simulink model "MySusp_StabiSystem_RTW"  (Simulink 10.3)
settings: Solver=ode1  StartTime=0.0  StopTime=inf  FixedStep=0.001  RelTol=1e-3
PreLoadFcn:
  | vehicle = 'Car'; if ~length(which('cmself')), cmenv; end
  | MySusp_StabiSystem_RTW_bus
  | MySusp_StabiSystem_RTW_params
InitFcn:
  | vehicle = 'Car'; if ~length(which('cmself')), cmenv; end
  | MySusp_StabiSystem_RTW_bus
undefined symbols (not defined in the file): Stiffness_F, Stiffness_R
Description:
  | CarMaker Plug-in Model Target
settings Model: Creator=ml  ModifiedByFormat=IPG  LastModifiedBy=IPG  MultithreadedSim=on
settings DataIOCC: SaveFormat=Dataset  SignalLoggingSaveFormat=Dataset  ReturnWorkspaceOutputs=on
settings OptimizationCC: ExpressionDepthLimit=128  LifeSpan=auto
settings DebuggingCC: UnderspecifiedInitializationDetection=Simplified  MergeDetectMultiDrivingBlocksExec=error  FcnCallInpInsideContextMsg=error  StateNameClashWarn=none  SFUnexpectedBacktrackingDiag=error  SFNoUnconditionalDefaultTransitionDiag=error  SFExecutionAtInitializationDiag=warning  SFMachineParentedDataDiag=error  ArithmeticOperatorsInVariantConditions=error
settings HardwareCC: ProdBitPerPointer=64  ProdBitPerSizeT=64  ProdBitPerPtrDiffT=64  ProdLargestAtomicFloat=Float  ProdIntDivRoundTo=Zero  ProdEndianess=LittleEndian  ProdWordSize=64  ProdHWDeviceType=Intel->x86-64 (Windows64)
settings ModelReferenceCC: PropagateSignalLabelsOutOfModel=on
settings SFSimCC: SimUseLocalCustomCode=on  CustomCodeUndefinedFunction=FilterOut
settings RTWCC: Description=CarMaker Plug-in Model Target  SystemTargetFile=CarMaker.tlc  TemplateMakefile=CarMaker_unix-win64.tmf  RTWUseLocalCustomCode=on
settings CodeAppCC: MaxIdLength=127  StateflowObjectComments=off
settings STFCustomTargetCC: TargetLangStandard=C99 (ISO)  CombineOutputUpdateFcns=on  MatFileLogging=on  CodeInterfacePackaging=Reusable function  GRTInterface=off  GenerateAllocFcn=on  SystemTargetFile=CarMaker.tlc
settings GRTTargetCC: TargetLangStandard=C99 (ISO)  ParMdlRefBuildCompliant=off  CompOptLevelCompliant=off  ConcurrentExecutionCompliant=off  CombineOutputUpdateFcns=on  CodeInterfacePackaging=Reusable function  CPPClassGenCompliant=off  GRTInterface=off  GenerateAllocFcn=on  UseToolchainInfoCompliant=off
settings CustomProperty: DataType=string
settings EnumStrPairs: String=Car
settings ConfigComp: CovMetricSettings=dwe  CovSaveCumulativeToWorkspaceVar=off  CovSaveSingleToWorkspaceVar=off  CovExternalEMLEnable=on

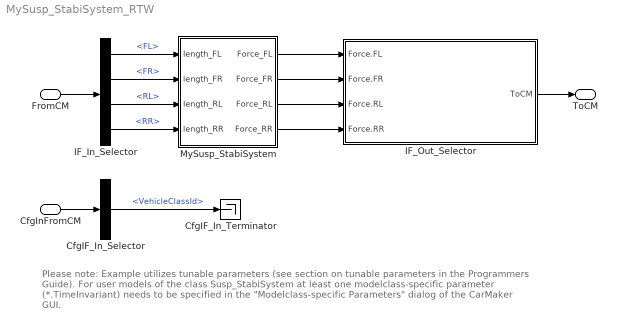
== system MySusp_StabiSystem_RTW ==
  note: Please note: Example utilizes tunable parameters (see section on tunable parameters in the Programmers Guide).
      |
      | For user models of the class Susp_StabiSystem at least one modelclass-specific parameter (*.TimeInvariant) needs to be
      | specified in the "Modelclass-specific Parameters" dialog of the CarMaker GUI.
  FromCM : Inport  OutDataTypeStr=Bus: cmSusp_StabiSystemIn
  CfgInFromCM : Inport  Port=2  OutDataTypeStr=Bus: cmSusp_StabiSystemCfgIn
  CfgIF_In_Selector : BusSelector  OutputSignals=VehicleClassId
  CfgIF_In_Terminator : Terminator
  IF_In_Selector : BusSelector  OutputSignals=length.FL,length.FR,length.RL,length.RR
  IF_Out_Selector : Subsystem  mask(Signal Selection){}
      mask help: Signal Selection Block
      settings: OpenFcn=cmSignalSelect('SignalSelection_CB',gcb)
  MySusp_StabiSystem : Subsystem
  ToCM : Outport  OutDataTypeStr=Bus: cmSusp_StabiSystemOut
  wires:
  FromCM/1 -> IF_In_Selector/1
  IF_Out_Selector/1(ToCM) -> ToCM/1
  CfgInFromCM/1 -> CfgIF_In_Selector/1
  CfgIF_In_Selector/1 -> CfgIF_In_Terminator/1  "<VehicleClassId>"
  MySusp_StabiSystem/1(Force_FL) -> IF_Out_Selector/1(Force.FL)
  MySusp_StabiSystem/2(Force_FR) -> IF_Out_Selector/2(Force.FR)
  MySusp_StabiSystem/3(Force_RL) -> IF_Out_Selector/3(Force.RL)
  MySusp_StabiSystem/4(Force_RR) -> IF_Out_Selector/4(Force.RR)
  IF_In_Selector/1 -> MySusp_StabiSystem/1(Iength_FL)  "<FL>"
  IF_In_Selector/2 -> MySusp_StabiSystem/2(length_FR)  "<FR>"
  IF_In_Selector/3 -> MySusp_StabiSystem/3(Iength_RL)  "<RL>"
  IF_In_Selector/4 -> MySusp_StabiSystem/4(length_RR)  "<RR>"

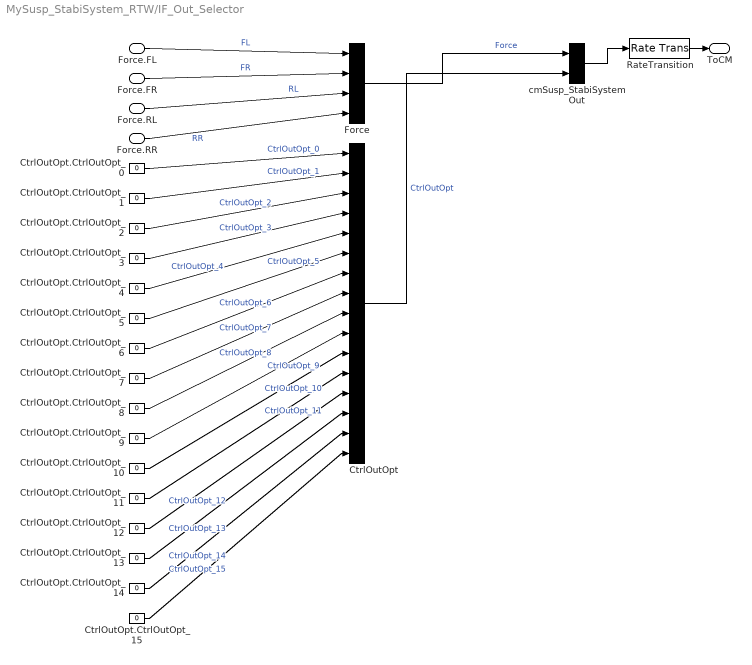
== system MySusp_StabiSystem_RTW/IF_Out_Selector ==
  Force.FL : Inport
  Force.FR : Inport  Port=2
  Force.RL : Inport  Port=3
  Force.RR : Inport  Port=4
  CtrlOutOpt : BusCreator  Inputs=16
  CtrlOutOpt.CtrlOutOpt_{0..15} (16 alike) : Constant  Value=0
  Force : BusCreator  Inputs=4
  RateTransition : RateTransition  OutPortSampleTime=str2num(get_param(bdroot,'FixedStep'))
  cmSusp_StabiSystemOut : BusCreator  Inputs=2
  ToCM : Outport
  wires:
  RateTransition/1 -> ToCM/1
  cmSusp_StabiSystemOut/1 -> RateTransition/1
  Force/1 -> cmSusp_StabiSystemOut/1  "Force"
  CtrlOutOpt/1 -> cmSusp_StabiSystemOut/2  "CtrlOutOpt"
  CtrlOutOpt.CtrlOutOpt_0/1 -> CtrlOutOpt/1  "CtrlOutOpt_0"
  CtrlOutOpt.CtrlOutOpt_1/1 -> CtrlOutOpt/2  "CtrlOutOpt_1"
  CtrlOutOpt.CtrlOutOpt_2/1 -> CtrlOutOpt/3  "CtrlOutOpt_2"
  CtrlOutOpt.CtrlOutOpt_3/1 -> CtrlOutOpt/4  "CtrlOutOpt_3"
  CtrlOutOpt.CtrlOutOpt_4/1 -> CtrlOutOpt/5  "CtrlOutOpt_4"
  CtrlOutOpt.CtrlOutOpt_5/1 -> CtrlOutOpt/6  "CtrlOutOpt_5"
  CtrlOutOpt.CtrlOutOpt_6/1 -> CtrlOutOpt/7  "CtrlOutOpt_6"
  CtrlOutOpt.CtrlOutOpt_7/1 -> CtrlOutOpt/8  "CtrlOutOpt_7"
  CtrlOutOpt.CtrlOutOpt_8/1 -> CtrlOutOpt/9  "CtrlOutOpt_8"
  CtrlOutOpt.CtrlOutOpt_9/1 -> CtrlOutOpt/10  "CtrlOutOpt_9"
  CtrlOutOpt.CtrlOutOpt_10/1 -> CtrlOutOpt/11  "CtrlOutOpt_10"
  CtrlOutOpt.CtrlOutOpt_11/1 -> CtrlOutOpt/12  "CtrlOutOpt_11"
  CtrlOutOpt.CtrlOutOpt_12/1 -> CtrlOutOpt/13  "CtrlOutOpt_12"
  CtrlOutOpt.CtrlOutOpt_13/1 -> CtrlOutOpt/14  "CtrlOutOpt_13"
  CtrlOutOpt.CtrlOutOpt_14/1 -> CtrlOutOpt/15  "CtrlOutOpt_14"
  CtrlOutOpt.CtrlOutOpt_15/1 -> CtrlOutOpt/16  "CtrlOutOpt_15"
  Force.FL/1 -> Force/1  "FL"
  Force.FR/1 -> Force/2  "FR"
  Force.RL/1 -> Force/3  "RL"
  Force.RR/1 -> Force/4  "RR"

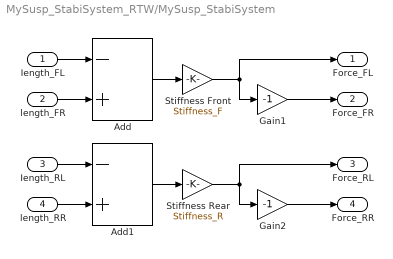
== system MySusp_StabiSystem_RTW/MySusp_StabiSystem ==
  Iength_FL : Inport
  length_FR : Inport  Port=2
  Iength_RL : Inport  Port=3
  length_RR : Inport  Port=4
  Add : Sum  Inputs=-+
  Add1 : Sum  Inputs=-+
  Gain1 : Gain  Gain=-1
  Gain2 : Gain  Gain=-1
  Stiffness Front : Gain  Gain=Stiffness_F
  Stiffness Rear : Gain  Gain=Stiffness_R
  Force_FL : Outport  VectorParamsAs1DForOutWhenUnconnected=off
  Force_FR : Outport  Port=2  VectorParamsAs1DForOutWhenUnconnected=off
  Force_RL : Outport  Port=3  VectorParamsAs1DForOutWhenUnconnected=off
  Force_RR : Outport  Port=4  VectorParamsAs1DForOutWhenUnconnected=off
  wires:
  Stiffness Front/1 -> Force_FL/1, Gain1/1
  Gain1/1 -> Force_FR/1
  Iength_FL/1 -> Add/1
  length_FR/1 -> Add/2
  Add/1 -> Stiffness Front/1
  Gain2/1 -> Force_RR/1
  Add1/1 -> Stiffness Rear/1
  Stiffness Rear/1 -> Force_RL/1, Gain2/1
  Iength_RL/1 -> Add1/1
  length_RR/1 -> Add1/2
